simulink model "csc_fps_feature_sensor_prep_hrn"  (R2014b)
settings: Solver=FixedStepDiscrete  StartTime=0  StopTime=12  FixedStep=1  RelTol=1e-3
libraries: csc_fps_feature_sensor_prep_lib x1
settings Model: Creator=escrane  LastModifiedBy=mstewart
settings DataIOCC: SignalLoggingSaveFormat=ModelDataLogs
settings OptimizationCC: ExpressionDepthLimit=2147483647
settings DebuggingCC: UnderspecifiedInitializationDetection=Classic  MergeDetectMultiDrivingBlocksExec=none  FcnCallInpInsideContextMsg=EnableAllAsWarning  StateNameClashWarn=warning

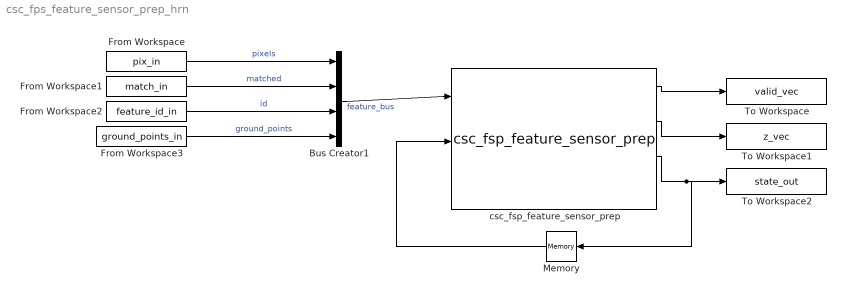
== system csc_fps_feature_sensor_prep_hrn ==
  Bus Creator1 : BusCreator
  From Workspace : FromWorkspace  VariableName=pix_in  SampleTime=0
  From Workspace1 : FromWorkspace  VariableName=match_in  SampleTime=0
  From Workspace2 : FromWorkspace  VariableName=feature_id_in  SampleTime=0
  From Workspace3 : FromWorkspace  VariableName=ground_points_in  SampleTime=0
  Memory : Memory  X0=zeros(24,1)  InheritSampleTime=on
  To Workspace : ToWorkspace  VariableName=valid_vec  SaveFormat=Timeseries  SampleTime=-1
  To Workspace1 : ToWorkspace  VariableName=z_vec  SaveFormat=Timeseries  SampleTime=-1
  To Workspace2 : ToWorkspace  VariableName=state_out  SaveFormat=Timeseries  SampleTime=-1
  csc_fsp_feature_sensor_prep : csc_fps_feature_sensor_prep_lib/csc_fsp_feature_sensor_prep
  wires:
  csc_fsp_feature_sensor_prep/1 -> To Workspace/1
  csc_fsp_feature_sensor_prep/2 -> To Workspace1/1
  From Workspace/1 -> Bus Creator1/1  "pixels"
  From Workspace1/1 -> Bus Creator1/2  "matched"
  Bus Creator1/1 -> csc_fsp_feature_sensor_prep/1  "feature_bus"
  From Workspace3/1 -> Bus Creator1/4  "ground_points"
  From Workspace2/1 -> Bus Creator1/3  "id"
  Memory/1 -> csc_fsp_feature_sensor_prep/2
  csc_fsp_feature_sensor_prep/3 -> Memory/1, To Workspace2/1
